simulink model "lab6"  (R2016a)
settings: Solver=VariableStepAuto  StartTime=0.0  StopTime=1  RelTol=1e-3
libraries: dsparch4 x1
settings Model: Creator=MMJ  LastModifiedBy=MMJ

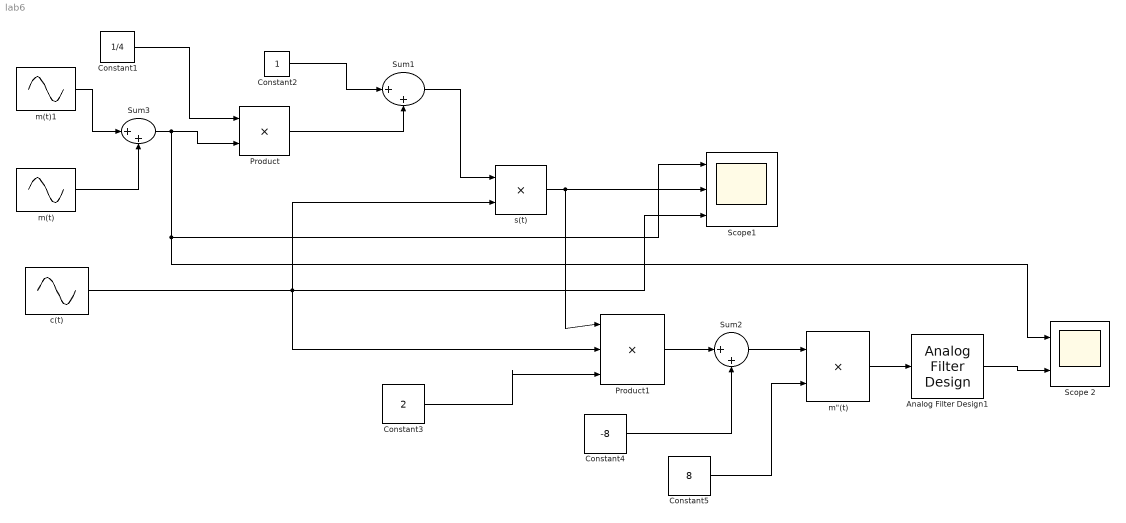
== system lab6 ==
  Analog Filter Design1 : dsparch4/Analog Filter Design  method=Butterworth  filttype=Lowpass  N=8  Wlo=2*pi*12  Whi=80  Rp=2  Rs=40
  Constant1 : Constant  Value=1/4
  Constant2 : Constant
  Constant3 : Constant  Value=2
  Constant4 : Constant  Value=-8
  Constant5 : Constant  Value=8
  Product : Product
  Product1 : Product  Inputs=3
  Scope 2 : Scope  NumInputPorts=2
  Scope1 : Scope  NumInputPorts=3
  Sum1 : Sum  Inputs=|++
  Sum2 : Sum  Inputs=|++
  Sum3 : Sum  Inputs=|++
  c(t) : Sin  Amplitude=2  Frequency=2*pi*50  Phase=pi/2  SampleTime=1/5000
  "m\"(t)" : Product
  m(t) : Sin  Amplitude=2  Frequency=2*pi*4  SampleTime=0
  m(t)1 : Sin  Amplitude=3  Frequency=2*pi*6  Phase=pi/2  SampleTime=0
  s(t) : Product
  wires:
  Constant1/1 -> Product/1
  Product/1 -> Sum1/2
  Constant2/1 -> Sum1/1
  Sum1/1 -> s(t)/1
  c(t)/1 -> s(t)/2, Scope1/3, Product1/2
  s(t)/1 -> Scope1/2, Product1/1
  Constant3/1 -> Product1/3
  Product1/1 -> Sum2/1
  Constant4/1 -> Sum2/2
  Constant5/1 -> "m\"(t)"/2
  Sum2/1 -> "m\"(t)"/1
  "m\"(t)"/1 -> Analog Filter Design1/1
  m(t)1/1 -> Sum3/1
  m(t)/1 -> Sum3/2
  Sum3/1 -> Scope 2/1, Scope1/1, Product/2
  Analog Filter Design1/1 -> Scope 2/2
